simulink model "Pacemaker_Deliverable_1"  (R2025a)
settings: Solver=FixedStepAuto  StartTime=0.0  StopTime=10.0  FixedStep=1e-3  RelTol=1e-3  EnableMultiTasking=on
undefined symbols (not defined in the file): D0, D1, D10, D11, D12, D13, D2, D3, D4, D5, D6, D7, D8, D9, PTA0, PTA1, PTA2, PTB23, PTB9, PTC16, PTC17, PTC2, PTC3, PTC4, PTD0, PTD1, PTD2, PTD3
libraries: frdmk64flib x14
settings Model: ExtModeTrigDuration=5  Creator=School Account  LastModifiedBy=user
settings SolverCC: AlgebraicLoopSolver=TrustRegion
settings OptimizationCC: DefaultParameterBehavior=Inlined  EnhancedBackFolding=on  PassReuseOutputArgsAs=Individual arguments  ZeroExternalMemoryAtStartup=off  ZeroInternalMemoryAtStartup=off  MaxStackSize=64  OptimizeBlockOrder=speed  DifferentSizesBufferReuse=on  OptimizationCustomize=off  EfficientTunableParamExpr=on
settings DebuggingCC: ParameterTunabilityLossMsg=error
settings HardwareCC: ProdBitPerPointer=32.0  ProdBitPerSizeT=32.0  ProdBitPerPtrDiffT=32.0  ProdLargestAtomicInteger=Long  ProdLargestAtomicFloat=Double  ProdWordSize=32.0  ProdHWDeviceType=ARM Compatible->ARM Cortex
settings SFSimCC: MATLABDynamicMemAlloc=off
settings RTWCC: SystemTargetFile=ert.tlc  HardwareBoard=NXP FRDM-K64F  TLCOptions="-aInlineSetEventsForThisBaseRateFcn=TLC_FALSE -aSuppressMultiTaskScheduler=TLC_FALSE  -aRateBasedStepFcn=0"  TemplateMakefile=ert_default_tmf  Toolchain=GNU Tools for ARM Embedded Processors  GPUComputeCapability=3.5  Description=Embedded Coder
settings CodeAppCC: ForceParamTrailComments=on  IgnoreCustomStorageClasses=off  OperatorAnnotations=on  SimulinkDataObjDesc=on  SFDataObjDesc=on  InsertBlockDesc=on
settings ERTTargetCC: ExtModeTransport=4.0  ExtModeStaticAlloc=off  ExtModeMexFile=sendToCommService  ExtModeIntrfLevel=Level1  DynamicArrayContainerType=coder::array

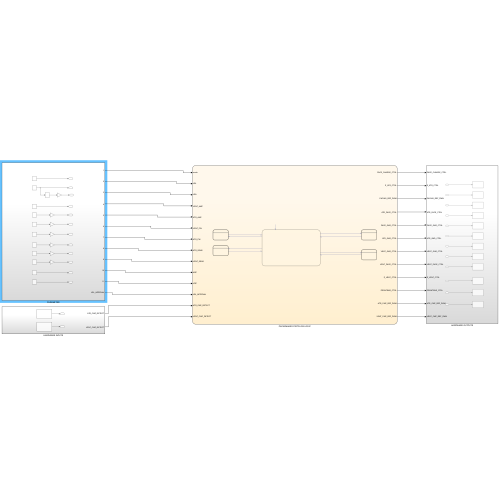
[thumbnail: Simulink's stored preview of the top-level diagram]
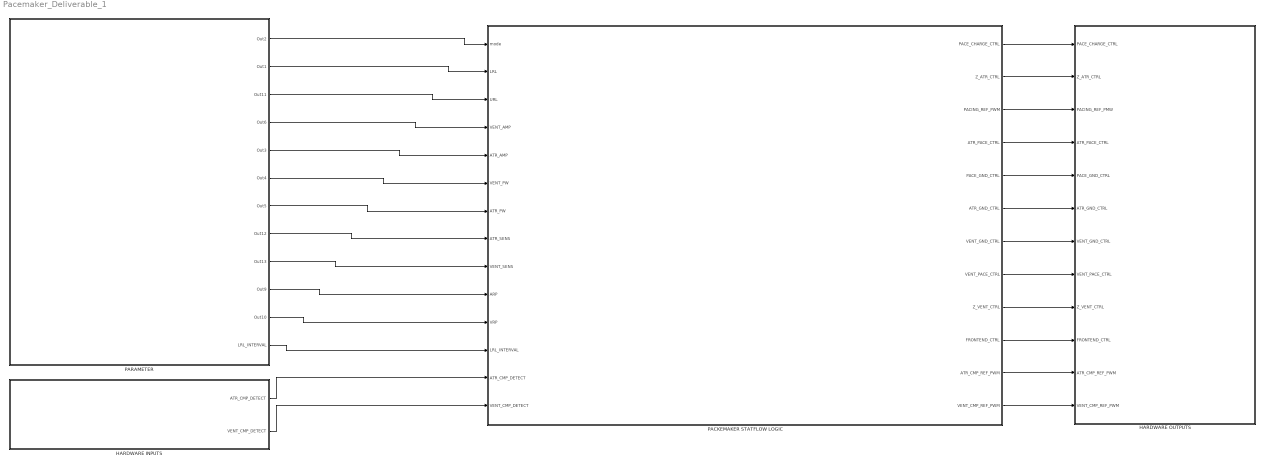
== system Pacemaker_Deliverable_1 ==
  HARDWARE INPUTS : Subsystem
  HARDWARE OUTPUTS : Subsystem
  PACKEMAKER STATFLOW LOGIC : Stateflow chart  TreatAsAtomicUnit=on
      settings: PortSchema="{\"entries\":[{\"content\":{\"sides\":[{\"content\":{\"connectorIds\":[\"In1\",\"In4\",\"In13\",\"In5\",\"In2\",\"In6\",\"In3\",\"In7\",\"In10\",\"In8\",\"In11\",\"In14\",\"In9\",\"In12\"]},\"type\":\"ConnectorPlacement.EquallySpacedRectSide\",\"uuid\":\"2821f65a-9b3e-4ca7-babd-b0602bfdca31\"},{\"content\":{\"connectorIds\":[\"Out1\",\"Out2\",\"Out3\",\"Out4\",\"Out5\",\"Out6\",\"Out7\",\"Out8\",\"Out9\",\"Out10\",\"Out11\",\"Out12\"],\"side\":\"RIGHT\"},\"type\":\"ConnectorPlacement.EquallySpacedRectSide\",\"uuid\":\"3302ad84-7e85-4bae-9388-240b69681e7f\"},{\"content\":{\"side\":\"TOP\"},\"type\":\"ConnectorPlacement.EquallySpacedRectSide\",\"uuid\":\"cc666da6-1c79-42dc-9f95-9791247ae8bf\"}]},\"type\":\"ConnectorPlacement.EquallySpacedConnector\",\"uuid\":\"e2a43bfa-d126-4f35-adbf-2cf33da0501f\"}],\"packageUris\":[\"http://schema.mathworks.com/mf0/Connector/R2020b\"],\"version\":\"1.0\"}"
  "PARAMETER " : Subsystem
  wires:
  PACKEMAKER STATFLOW LOGIC/1(PACE_CHARGE_CTRL) -> HARDWARE OUTPUTS/1(PACE_CHARGE_CTRL)
  PACKEMAKER STATFLOW LOGIC/2(Z_ATR_CTRL) -> HARDWARE OUTPUTS/2(Z_ATR_CTRL)
  PACKEMAKER STATFLOW LOGIC/3(PACING_REF_PWM) -> HARDWARE OUTPUTS/3(PACING_REF_PMW)
  PACKEMAKER STATFLOW LOGIC/4(ATR_PACE_CTRL) -> HARDWARE OUTPUTS/4(ATR_PACE_CTRL)
  PACKEMAKER STATFLOW LOGIC/5(PACE_GND_CTRL) -> HARDWARE OUTPUTS/5(PACE_GND_CTRL)
  PACKEMAKER STATFLOW LOGIC/6(ATR_GND_CTRL) -> HARDWARE OUTPUTS/6(ATR_GND_CTRL)
  PACKEMAKER STATFLOW LOGIC/7(VENT_GND_CTRL) -> HARDWARE OUTPUTS/7(VENT_GND_CTRL)
  PACKEMAKER STATFLOW LOGIC/8(VENT_PACE_CTRL) -> HARDWARE OUTPUTS/8(VENT_PACE_CTRL)
  PACKEMAKER STATFLOW LOGIC/9(Z_VENT_CTRL) -> HARDWARE OUTPUTS/9(Z_VENT_CTRL)
  PACKEMAKER STATFLOW LOGIC/10(FRONTEND_CTRL) -> HARDWARE OUTPUTS/10(FRONTEND_CTRL)
  PACKEMAKER STATFLOW LOGIC/11(ATR_CMP_REF_PWM) -> HARDWARE OUTPUTS/11(ATR_CMP_REF_PWM)
  PACKEMAKER STATFLOW LOGIC/12(VENT_CMP_REF_PWM) -> HARDWARE OUTPUTS/12(VENT_CMP_REF_PWM)
  HARDWARE INPUTS/2(VENT_CMP_DETECT) -> PACKEMAKER STATFLOW LOGIC/12(VENT_CMP_DETECT)
  HARDWARE INPUTS/1(ATR_CMP_DETECT) -> PACKEMAKER STATFLOW LOGIC/9(ATR_CMP_DETECT)
  "PARAMETER "/10(Out9) -> PACKEMAKER STATFLOW LOGIC/8(ARP)
  "PARAMETER "/11(Out10) -> PACKEMAKER STATFLOW LOGIC/11(VRP)
  "PARAMETER "/9(Out13) -> PACKEMAKER STATFLOW LOGIC/10(VENT_SENS)
  "PARAMETER "/8(Out12) -> PACKEMAKER STATFLOW LOGIC/7(ATR_SENS)
  "PARAMETER "/7(Out5) -> PACKEMAKER STATFLOW LOGIC/3(ATR_PW)
  "PARAMETER "/6(Out4) -> PACKEMAKER STATFLOW LOGIC/6(VENT_PW)
  "PARAMETER "/5(Out3) -> PACKEMAKER STATFLOW LOGIC/2(ATR_AMP)
  "PARAMETER "/4(Out6) -> PACKEMAKER STATFLOW LOGIC/5(VENT_AMP)
  "PARAMETER "/1(Out2) -> PACKEMAKER STATFLOW LOGIC/1(mode)
  "PARAMETER "/2(Out1) -> PACKEMAKER STATFLOW LOGIC/4(LRL)
  "PARAMETER "/3(Out11) -> PACKEMAKER STATFLOW LOGIC/13(URL)
  "PARAMETER "/12(LRL_INTERVAL) -> PACKEMAKER STATFLOW LOGIC/14(LRL_INTERVAL)

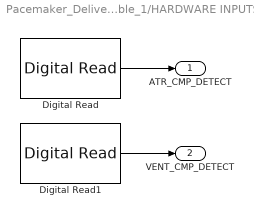
== system Pacemaker_Deliverable_1/HARDWARE INPUTS ==
  Digital Read : frdmk64flib/Digital Read  Whichpin=PTC16 (D0)  SampleTime=-1
  Digital Read1 : frdmk64flib/Digital Read  Whichpin=PTC17 (D1)  SampleTime=0.01
  ATR_CMP_DETECT : Outport
  VENT_CMP_DETECT : Outport  Port=2
  wires:
  Digital Read1/1 -> VENT_CMP_DETECT/1
  Digital Read/1 -> ATR_CMP_DETECT/1

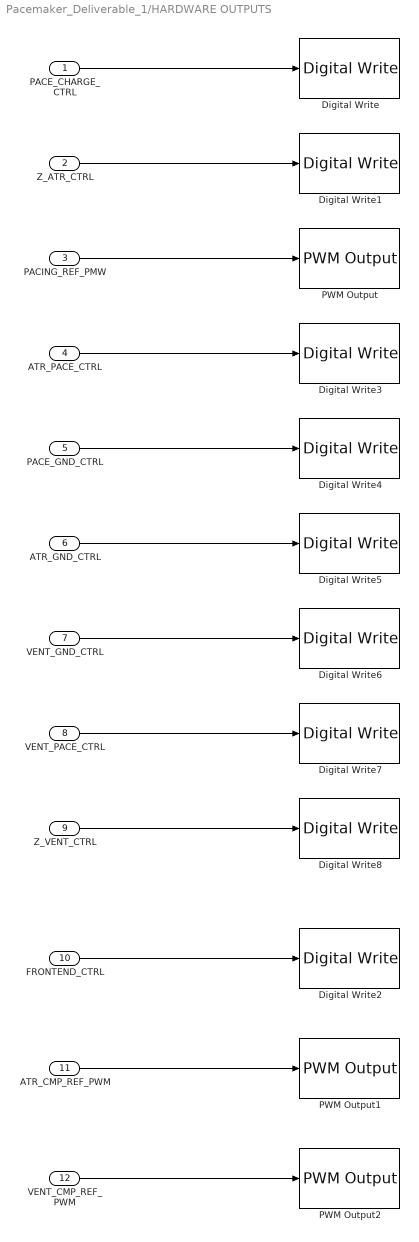
== system Pacemaker_Deliverable_1/HARDWARE OUTPUTS ==
  PACE_CHARGE_CTRL : Inport
  Z_ATR_CTRL : Inport  Port=2
  PACING_REF_PMW : Inport  Port=3
  ATR_PACE_CTRL : Inport  Port=4
  PACE_GND_CTRL : Inport  Port=5
  ATR_GND_CTRL : Inport  Port=6
  VENT_GND_CTRL : Inport  Port=7
  VENT_PACE_CTRL : Inport  Port=8
  Z_VENT_CTRL : Inport  Port=9
  FRONTEND_CTRL : Inport  Port=10
  ATR_CMP_REF_PWM : Inport  Port=11
  VENT_CMP_REF_PWM : Inport  Port=12
  Digital Write : frdmk64flib/Digital Write  Whichpin=PTB9 (D2)
  Digital Write1 : frdmk64flib/Digital Write  Whichpin=PTB23 (D4)
  Digital Write2 : frdmk64flib/Digital Write  Whichpin=PTD1 (D13)
  Digital Write3 : frdmk64flib/Digital Write  Whichpin=PTA0 (D8)
  Digital Write4 : frdmk64flib/Digital Write  Whichpin=PTD0 (D10)
  Digital Write5 : frdmk64flib/Digital Write  Whichpin=PTD2 (D11)
  Digital Write6 : frdmk64flib/Digital Write  Whichpin=PTD3 (D12)
  Digital Write7 : frdmk64flib/Digital Write  Whichpin=PTC4 (D9)
  Digital Write8 : frdmk64flib/Digital Write  Whichpin=PTC3 (D7)
  PWM Output : frdmk64flib/PWM Output  Whichpin=PTA2 (D5)  InitialFrequency=2000  InitialDutyCycle=0
  PWM Output1 : frdmk64flib/PWM Output  Whichpin=PTC2 (D6)  InitialFrequency=2000  InitialDutyCycle=0
  PWM Output2 : frdmk64flib/PWM Output  Whichpin=PTA1 (D3)  InitialFrequency=2000  InitialDutyCycle=0
  wires:
  PACE_CHARGE_CTRL/1 -> Digital Write/1
  Z_ATR_CTRL/1 -> Digital Write1/1
  PACING_REF_PMW/1 -> PWM Output/1
  ATR_PACE_CTRL/1 -> Digital Write3/1
  PACE_GND_CTRL/1 -> Digital Write4/1
  ATR_GND_CTRL/1 -> Digital Write5/1
  VENT_GND_CTRL/1 -> Digital Write6/1
  VENT_PACE_CTRL/1 -> Digital Write7/1
  Z_VENT_CTRL/1 -> Digital Write8/1
  FRONTEND_CTRL/1 -> Digital Write2/1
  ATR_CMP_REF_PWM/1 -> PWM Output1/1
  VENT_CMP_REF_PWM/1 -> PWM Output2/1

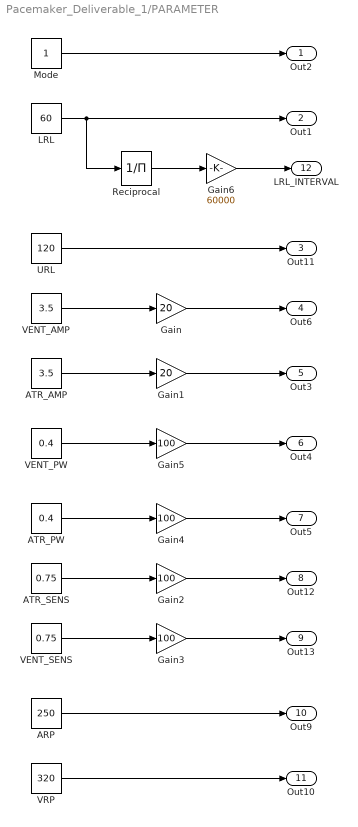
== system Pacemaker_Deliverable_1/PARAMETER  ==
  ARP : Constant  Value=250
  ATR_AMP : Constant  Value=3.5
  ATR_PW : Constant  Value=0.4
  ATR_SENS : Constant  Value=0.75
  Gain : Gain  Gain=20
  Gain1 : Gain  Gain=20
  Gain{2..5} (4 alike) : Gain  Gain=100
  Gain6 : Gain  Gain=60000
  LRL : Constant  Value=60
  Mode : Constant
  Reciprocal : Product  Inputs=/
  URL : Constant  Value=120
  VENT_AMP : Constant  Value=3.5
  VENT_PW : Constant  Value=0.4
  VENT_SENS : Constant  Value=0.75
  VRP : Constant  Value=320
  Out2 : Outport
  Out1 : Outport  Port=2
  Out11 : Outport  Port=3
  Out6 : Outport  Port=4
  Out3 : Outport  Port=5
  Out4 : Outport  Port=6
  Out5 : Outport  Port=7
  Out12 : Outport  Port=8
  Out13 : Outport  Port=9
  Out9 : Outport  Port=10
  Out10 : Outport  Port=11
  LRL_INTERVAL : Outport  Port=12
  wires:
  LRL/1 -> Reciprocal/1, Out1/1
  URL/1 -> Out11/1
  Mode/1 -> Out2/1
  ARP/1 -> Out9/1
  VRP/1 -> Out10/1
  VENT_AMP/1 -> Gain/1
  Gain/1 -> Out6/1
  ATR_AMP/1 -> Gain1/1
  Gain1/1 -> Out3/1
  ATR_SENS/1 -> Gain2/1
  Gain2/1 -> Out12/1
  VENT_SENS/1 -> Gain3/1
  Gain3/1 -> Out13/1
  VENT_PW/1 -> Gain5/1
  Gain5/1 -> Out4/1
  ATR_PW/1 -> Gain4/1
  Gain4/1 -> Out5/1
  Reciprocal/1 -> Gain6/1
  Gain6/1 -> LRL_INTERVAL/1

== stateflow chart Pacemaker_Deliverable_1/PACKEMAKER STATFLOW LOGIC ==
  state AAI
    state AAI_Charge
      entry:
      FRONTEND_CTRL = 1;
      %Charging C22
      ATR_PACE_CTRL = 0;
      VENT_PACE_CTRL = 0;
      PACING_REF_PWM = ATR_AMP;
      PACE_CHARGE_CTRL = 1;
      %Discharging C21
      PACE_GND_CTRL = 1;
      ATR_PACE_CTRL = 0;
      Z_VENT_CTRL = 0;
      Z_ATR_CTRL = 0;
      VENT_PACE_CTRL = 0;
      VENT_GND_CTRL = 0;
      ATR_GND_CTRL = 1;
      ATR_CMP_REF_PWM = ATR_SENS;
    state AAI_Pace
      entry:
      FRONTEND_CTRL = 0;
      %Pacing
      PACE_CHARGE_CTRL = 0;
      PACE_GND_CTRL= 1;
      VENT_PACE_CTRL = 0;
      VENT_GND_CTRL= 0;
      Z_VENT_CTRL = 0;
      Z_ATR_CTRL = 0;
      ATR_GND_CTRL = 0;
      ATR_PACE_CTRL= 1;
    (default) -> AAI_Charge
    AAI_Charge -> AAI_Pace [order 1] : [after(LRL_INTERVAL - ATR_PW - ARP,msec)]
    AAI_Pace -> AAI_Charge : [after(ATR_PW,msec)]
    (junction 58) -> (junction 84) : [after(ATR_PW,msec)]
    AAI_Charge -> (junction 58) [order 2] : [ATR_CMP_DETECT == 1]
    (junction 84) -> AAI_Charge : [after(ARP, msec)]
  state Start
  state VOO
    state VOO_Charge
      entry:
      %Charging C22
      VENT_PACE_CTRL = 0;
      ATR_PACE_CTRL = 0;
      PACING_REF_PWM = VENT_AMP;
      PACE_CHARGE_CTRL = 1;
      %Discharging C21
      PACE_GND_CTRL = 1;
      VENT_PACE_CTRL = 0;
      Z_ATR_CTRL = 0;
      Z_VENT_CTRL = 0;
      ATR_PACE_CTRL = 0;
      ATR_GND_CTRL = 0;
      VENT_GND_CTRL = 1;
    state AOO_Pace
      entry:
      %Pacing
      PACE_CHARGE_CTRL = 0;
      PACE_GND_CTRL= 1;
      ATR_PACE_CTRL = 0;
      ATR_GND_CTRL= 0;
      Z_ATR_CTRL = 0;
      Z_VENT_CTRL = 0;
      VENT_GND_CTRL = 0;
      VENT_PACE_CTRL = 1;
    (default) -> VOO_Charge
    VOO_Charge -> VOO.AOO_Pace : [after(LRL_INTERVAL - VENT_PW,msec)]
    VOO.AOO_Pace -> VOO_Charge : [after(VENT_PW,msec)]
  state AOO
    state AOO_Charge
      entry:
      %Charging C22
      ATR_PACE_CTRL = 0;
      VENT_PACE_CTRL = 0;
      PACING_REF_PWM = ATR_AMP;
      PACE_CHARGE_CTRL = 1;
      %Discharging C21
      PACE_GND_CTRL = 1;
      ATR_PACE_CTRL = 0;
      Z_VENT_CTRL = 0;
      Z_ATR_CTRL = 0;
      VENT_PACE_CTRL = 0;
      VENT_GND_CTRL = 0;
      ATR_GND_CTRL = 1;
    state AOO_Pace
      entry:
      %Pacing
      PACE_CHARGE_CTRL = 0;
      PACE_GND_CTRL= 1;
      VENT_PACE_CTRL = 0;
      VENT_GND_CTRL= 0;
      Z_VENT_CTRL = 0;
      Z_ATR_CTRL = 0;
      ATR_GND_CTRL = 0;
      ATR_PACE_CTRL = 1;
    (default) -> AOO_Charge
    AOO_Charge -> AOO.AOO_Pace : [after(LRL_INTERVAL - ATR_PW,msec)]
    AOO.AOO_Pace -> AOO_Charge : [after(ATR_PW,msec)]
  state VVI
    state VVI_Charge
      entry:
      FRONTEND_CTRL = 1;
      %Charging C22
      VENT_PACE_CTRL = 0;
      ATR_PACE_CTRL = 0;
      PACING_REF_PWM = VENT_AMP;
      PACE_CHARGE_CTRL = 1;
      %Discharging C21
      PACE_GND_CTRL = 1;
      VENT_PACE_CTRL = 0;
      Z_ATR_CTRL = 0;
      Z_VENT_CTRL = 0;
      ATR_PACE_CTRL = 0;
      ATR_GND_CTRL = 0;
      VENT_GND_CTRL = 1;
      VENT_CMP_REF_PWM = VENT_SENS;
    state VVI_Pace
      entry:
      FRONTEND_CTRL = 0;
      %Pacing
      PACE_CHARGE_CTRL = 0;
      PACE_GND_CTRL= 1;
      ATR_PACE_CTRL = 0;
      ATR_GND_CTRL= 0;
      Z_ATR_CTRL = 0;
      Z_VENT_CTRL = 0;
      VENT_GND_CTRL = 0;
      VENT_PACE_CTRL = 1;
    (default) -> VVI_Charge
    VVI_Charge -> VVI_Pace [order 1] : [after(LRL_INTERVAL - VENT_PW - VRP,msec)]
    VVI_Pace -> VVI_Charge [order 1] : [after(VENT_PW,msec)]
    VVI_Charge -> (junction 65) [order 2] : [VENT_CMP_DETECT == 1]
    (junction 65) -> (junction 82) : [after(VENT_PW,msec)]
    VVI_Pace -> (junction 82) [order 2] : [after(VENT_PW,msec)]
    (junction 82) -> VVI_Charge : [after(VRP, msec)]
  (default) -> Start
  Start -> VOO [order 1] : [mode == 2]
  AAI -> Start : [mode ~= 3]
  Start -> AAI [order 3] : [mode == 3]
  VOO -> Start : [mode ~= 2]
  Start -> AOO [order 2] : [mode == 1]
  AOO -> Start : [mode ~= 1]
  Start -> VVI [order 4] : [mode == 4]
  VVI -> Start : [mode ~= 4]
  data: PACE_CHARGE_CTRL output; Z_ATR_CTRL output; PACING_REF_PWM output; mode input; ATR_PACE_CTRL output; PACE_GND_CTRL output; ATR_AMP input; ATR_GND_CTRL output; ATR_PW input; LRL input; VENT_AMP input; VENT_GND_CTRL output; VENT_PACE_CTRL output; Z_VENT_CTRL output; VENT_PW input; FRONTEND_CTRL output; ATR_CMP_REF_PWM output; ATR_SENS input; ARP input; ATR_CMP_DETECT input; VENT_SENS input; VENT_CMP_REF_PWM output; VRP input; VENT_CMP_DETECT input; URL input; LRL_INTERVAL input
